simulink model "creating_fake_data"  (R2020b)
settings: Solver=VariableStepAuto  StartTime=0.0  StopTime=24  RelTol=1e-3
libraries: SignalEditorBlockLib x1
settings Model: Creator=Mostafa  LastModifiedBy=Mostafa

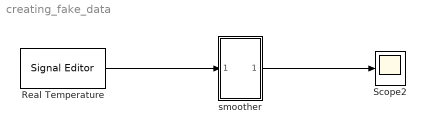
== system creating_fake_data ==
  Real Temperature : SignalEditorBlockLib/Signal Editor  FileName=fake_data_for_editor.mat  ActiveScenario=Scenario  ActiveSignal=Signal 1  IsBus=off  OutputBusObjectStr=Bus: BusObject  SampleTime=-1  ZeroCross=off  OutputAfterFinalValue=Holding final value  Unit=inherit  PreserveSignalName=on
  Scope2 : Scope
  smoother : Subsystem
  wires:
  Real Temperature/1 -> smoother/1(In1)
  smoother/1(Out1) -> Scope2/1

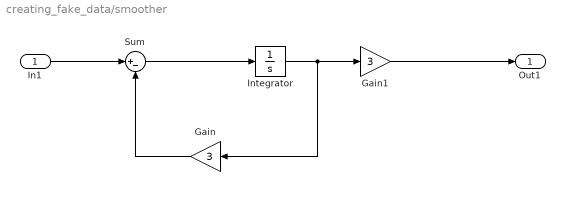
== system creating_fake_data/smoother ==
  In1 : Inport
  Gain : Gain  Gain=3
  Gain1 : Gain  Gain=3
  Integrator : Integrator  InitialCondition=24/3
  Sum : Sum  Inputs=|+-
  Out1 : Outport
  wires:
  Gain/1 -> Sum/2
  Sum/1 -> Integrator/1
  Gain1/1 -> Out1/1
  In1/1 -> Sum/1
  Integrator/1 -> Gain1/1, Gain/1
